simulink library "EOM_lib_incomplete"  (R2020a)
settings: Solver=VariableStepAuto  StartTime=0.0  StopTime=10.0  RelTol=1e-3
undefined symbols (not defined in the file or in its folder): g
libraries: $bdroot x1
settings Model: Creator=muril  LastModifiedBy=muril

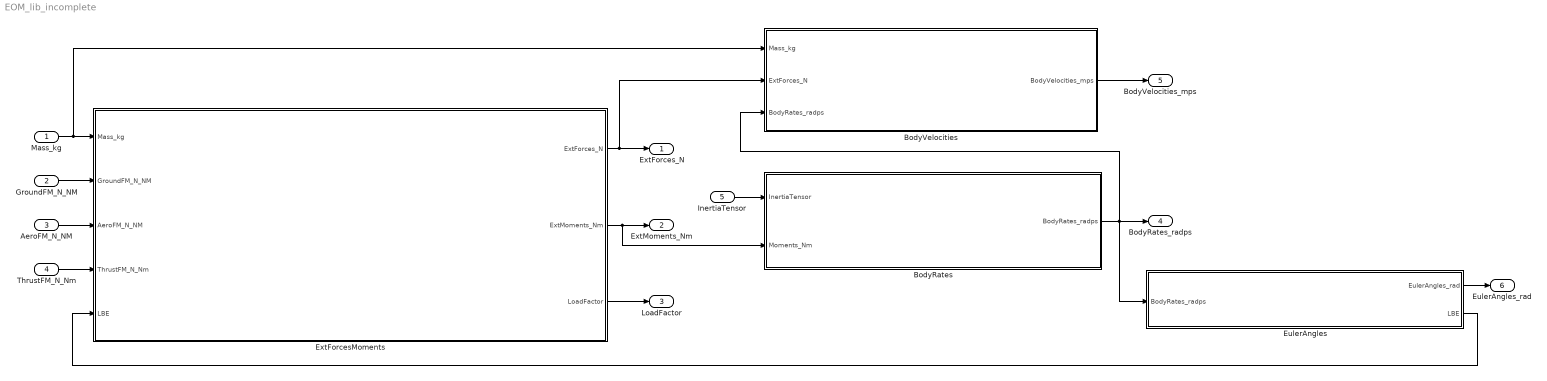
== system EOM_lib_incomplete ==
  Mass_kg : Inport
  GroundFM_N_NM : Inport  Port=2
  AeroFM_N_NM : Inport  Port=3
  ThrustFM_N_Nm : Inport  Port=4
  InertiaTensor : Inport  Port=5
  BodyRates : Subsystem
  BodyVelocities : Subsystem
  EulerAngles : Subsystem
  ExtForcesMoments : Subsystem
  ExtForces_N : Outport
  ExtMoments_Nm : Outport  Port=2
  LoadFactor : Outport  Port=3
  BodyRates_radps : Outport  Port=4
  BodyVelocities_mps : Outport  Port=5
  EulerAngles_rad : Outport  Port=6
  wires:
  EulerAngles/2(LBE) -> ExtForcesMoments/5(LBE)
  GroundFM_N_NM/1 -> ExtForcesMoments/2(GroundFM_N_NM)
  AeroFM_N_NM/1 -> ExtForcesMoments/3(AeroFM_N_NM)
  ThrustFM_N_Nm/1 -> ExtForcesMoments/4(ThrustFM_N_Nm)
  ExtForcesMoments/3(LoadFactor) -> LoadFactor/1
  InertiaTensor/1 -> BodyRates/1(InertiaTensor)
  ExtForcesMoments/2(ExtMoments_Nm) -> ExtMoments_Nm/1, BodyRates/2(Moments_Nm)
  BodyRates/1(BodyRates_radps) -> EulerAngles/1(BodyRates_radps), BodyRates_radps/1, BodyVelocities/3(BodyRates_radps)
  BodyVelocities/1(BodyVelocities_mps) -> BodyVelocities_mps/1
  ExtForcesMoments/1(ExtForces_N) -> BodyVelocities/2(ExtForces_N), ExtForces_N/1
  Mass_kg/1 -> BodyVelocities/1(Mass_kg), ExtForcesMoments/1(Mass_kg)
  EulerAngles/1(EulerAngles_rad) -> EulerAngles_rad/1

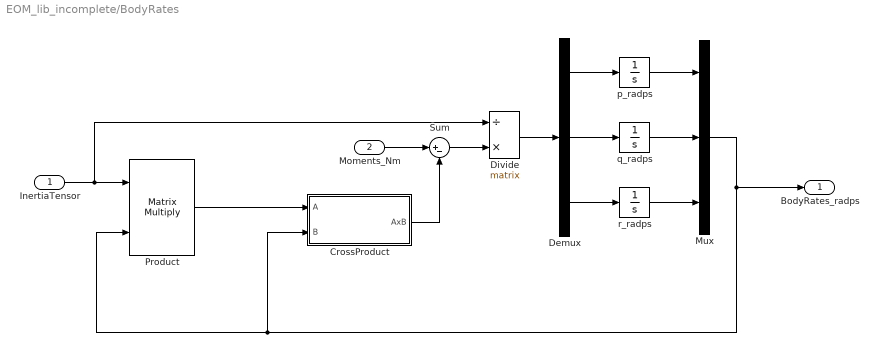
== system EOM_lib_incomplete/BodyRates ==
  InertiaTensor : Inport
  Moments_Nm : Inport  Port=2
  CrossProduct : Subsystem
  Demux : Demux  Outputs=3
  Divide : Product  Inputs=/*  Multiplication=Matrix(*)
  Mux : Mux  Inputs=3
  Product : Product  Multiplication=Matrix(*)
  Sum : Sum  Inputs=|+-
  p_radps : Integrator  ContinuousStateAttributes='p_radps'
  q_radps : Integrator  ContinuousStateAttributes='q_radps'
  r_radps : Integrator  ContinuousStateAttributes='r_radps'
  BodyRates_radps : Outport
  wires:
  Mux/1 -> BodyRates_radps/1, Product/2, CrossProduct/2(B)
  r_radps/1 -> Mux/3
  InertiaTensor/1 -> Product/1, Divide/1
  Product/1 -> CrossProduct/1(A)
  q_radps/1 -> Mux/2
  p_radps/1 -> Mux/1
  CrossProduct/1(AxB) -> Sum/2
  Demux/1 -> p_radps/1
  Sum/1 -> Divide/2
  Divide/1 -> Demux/1
  Moments_Nm/1 -> Sum/1
  Demux/2 -> q_radps/1
  Demux/3 -> r_radps/1

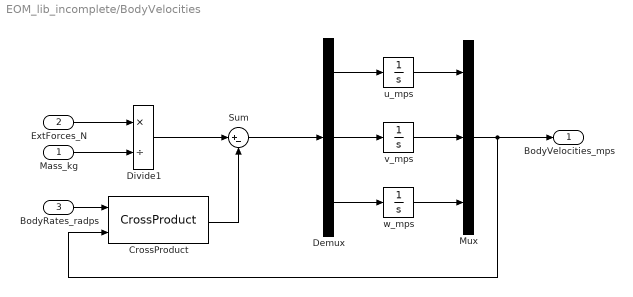
== system EOM_lib_incomplete/BodyVelocities ==
  Mass_kg : Inport
  ExtForces_N : Inport  Port=2
  BodyRates_radps : Inport  Port=3
  CrossProduct : $bdroot/BodyRates/CrossProduct  SystemSampleTime=-1  Latency=0  AutoFrameSizeCalculation=off
  Demux : Demux  Outputs=3
  Divide1 : Product  Inputs=*/
  Mux : Mux  Inputs=3
  Sum : Sum  Inputs=|+-
  u_mps : Integrator  ContinuousStateAttributes='u_mps'
  v_mps : Integrator  ContinuousStateAttributes='v_mps'
  w_mps : Integrator  ContinuousStateAttributes='w_mps'
  BodyVelocities_mps : Outport
  wires:
  BodyRates_radps/1 -> CrossProduct/1
  CrossProduct/1 -> Sum/2
  Demux/2 -> v_mps/1
  Demux/3 -> w_mps/1
  Divide1/1 -> Sum/1
  Demux/1 -> u_mps/1
  w_mps/1 -> Mux/3
  Mux/1 -> BodyVelocities_mps/1, CrossProduct/2
  u_mps/1 -> Mux/1
  Sum/1 -> Demux/1
  v_mps/1 -> Mux/2
  ExtForces_N/1 -> Divide1/1
  Mass_kg/1 -> Divide1/2

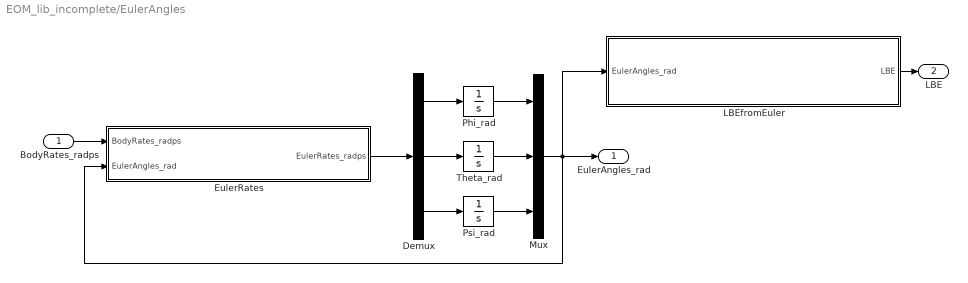
== system EOM_lib_incomplete/EulerAngles ==
  BodyRates_radps : Inport
  Demux : Demux  Outputs=3
  EulerRates : Subsystem
  LBEfromEuler : Subsystem
  Mux : Mux  Inputs=3
  Phi_rad : Integrator  ContinuousStateAttributes='Phi_rad'
  Psi_rad : Integrator  ContinuousStateAttributes='Psi_rad'
  Theta_rad : Integrator  ContinuousStateAttributes='Theta_rad'
  EulerAngles_rad : Outport
  LBE : Outport  Port=2
  wires:
  BodyRates_radps/1 -> EulerRates/1(BodyRates_radps)
  Demux/3 -> Psi_rad/1
  Theta_rad/1 -> Mux/2
  Psi_rad/1 -> Mux/3
  Mux/1 -> EulerRates/2(EulerAngles_rad), EulerAngles_rad/1, LBEfromEuler/1(EulerAngles_rad)
  Demux/1 -> Phi_rad/1
  Demux/2 -> Theta_rad/1
  Phi_rad/1 -> Mux/1
  EulerRates/1(EulerRates_radps) -> Demux/1
  LBEfromEuler/1(LBE) -> LBE/1

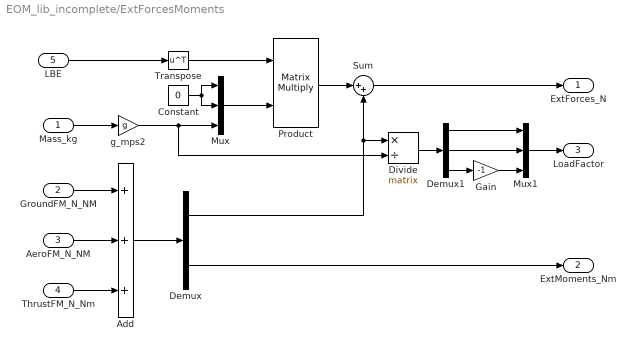
== system EOM_lib_incomplete/ExtForcesMoments ==
  Mass_kg : Inport
  GroundFM_N_NM : Inport  Port=2
  AeroFM_N_NM : Inport  Port=3
  ThrustFM_N_Nm : Inport  Port=4
  LBE : Inport  Port=5
  Add : Sum  Inputs=+++
  Constant : Constant  Value=0
  Demux : Demux  Outputs=2
  Demux1 : Demux  Outputs=3
  Divide : Product  Inputs=*/  Multiplication=Matrix(*)
  Gain : Gain  Gain=-1
  Mux : Mux  Inputs=3
  Mux1 : Mux  Inputs=3
  Product : Product  Multiplication=Matrix(*)
  Sum : Sum  Inputs=|++
  Transpose : Math  Operator=transpose  SaturateOnIntegerOverflow=on
  g_mps2 : Gain  Gain=g
  ExtForces_N : Outport
  ExtMoments_Nm : Outport  Port=2
  LoadFactor : Outport  Port=3
  wires:
  Demux/2 -> ExtMoments_Nm/1
  AeroFM_N_NM/1 -> Add/2
  Mux1/1 -> LoadFactor/1
  Constant/1 -> Mux/1, Mux/2
  Gain/1 -> Mux1/3
  Sum/1 -> ExtForces_N/1
  Demux/1 -> Divide/1, Sum/2
  ThrustFM_N_Nm/1 -> Add/3
  g_mps2/1 -> Divide/2, Mux/3
  GroundFM_N_NM/1 -> Add/1
  Add/1 -> Demux/1
  LBE/1 -> Transpose/1
  Demux1/3 -> Gain/1
  Mux/1 -> Product/2
  Mass_kg/1 -> g_mps2/1
  Transpose/1 -> Product/1
  Demux1/1 -> Mux1/1
  Product/1 -> Sum/1
  Demux1/2 -> Mux1/2
  Divide/1 -> Demux1/1

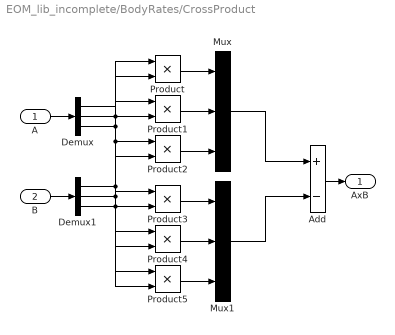
== system EOM_lib_incomplete/BodyRates/CrossProduct ==
  A : Inport
  B : Inport  Port=2
  Add : Sum  Inputs=+-
  Demux : Demux  Outputs=3
  Demux1 : Demux  Outputs=3
  Mux : Mux  Inputs=3
  Mux1 : Mux  Inputs=3
  Product{,1..5} (6 alike) : Product
  AxB : Outport
  wires:
  Demux1/1 -> Product5/2, Product1/2
  Mux1/1 -> Add/2
  Product1/1 -> Mux/2
  Product5/1 -> Mux1/3
  Demux/1 -> Product2/1, Product4/1
  Demux/3 -> Product3/1, Product1/1
  Demux/2 -> Product5/1, Product/1
  Demux1/2 -> Product3/2, Product2/2
  Product2/1 -> Mux/3
  A/1 -> Demux/1
  Product3/1 -> Mux1/1
  Add/1 -> AxB/1
  Demux1/3 -> Product4/2, Product/2
  Product/1 -> Mux/1
  Product4/1 -> Mux1/2
  Mux/1 -> Add/1
  B/1 -> Demux1/1

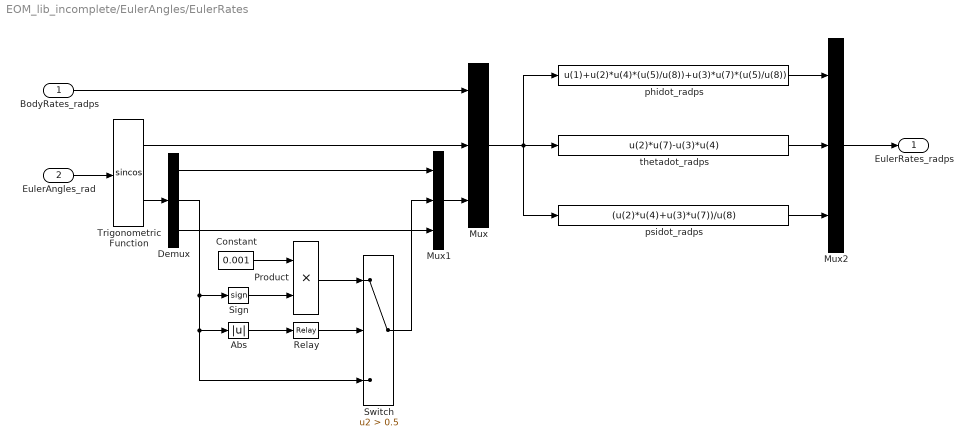
== system EOM_lib_incomplete/EulerAngles/EulerRates ==
  BodyRates_radps : Inport
  EulerAngles_rad : Inport  Port=2
  Abs : Abs
  Constant : Constant  Value=0.001
  Demux : Demux  Outputs=3
  Mux : Mux  Inputs=3
  Mux1 : Mux  Inputs=3
  Mux2 : Mux  Inputs=3
  Product : Product
  Relay : Relay  OnSwitchValue=0.001  OffSwitchValue=0  OnOutputValue=0  OffOutputValue=1
  Sign : Signum
  Switch : Switch  Criteria=u2 > Threshold  Threshold=0.5
  Trigonometric Function : Trigonometry  Operator=sincos
  phidot_radps : Fcn  Expr=u(1)+u(2)*u(4)*(u(5)/u(8))+u(3)*u(7)*(u(5)/u(8))
  psidot_radps : Fcn  Expr=(u(2)*u(4)+u(3)*u(7))/u(8)
  thetadot_radps : Fcn  Expr=u(2)*u(7)-u(3)*u(4)
  EulerRates_radps : Outport
  wires:
  Demux/3 -> Mux1/3
  Mux/1 -> psidot_radps/1, thetadot_radps/1, phidot_radps/1
  Trigonometric Function/1 -> Mux/2
  Mux2/1 -> EulerRates_radps/1
  BodyRates_radps/1 -> Mux/1
  Constant/1 -> Product/1
  Trigonometric Function/2 -> Demux/1
  Product/1 -> Switch/1
  EulerAngles_rad/1 -> Trigonometric Function/1
  psidot_radps/1 -> Mux2/3
  Demux/2 -> Abs/1, Switch/3, Sign/1
  Abs/1 -> Relay/1
  Demux/1 -> Mux1/1
  phidot_radps/1 -> Mux2/1
  Sign/1 -> Product/2
  Mux1/1 -> Mux/3
  Switch/1 -> Mux1/2
  Relay/1 -> Switch/2
  thetadot_radps/1 -> Mux2/2

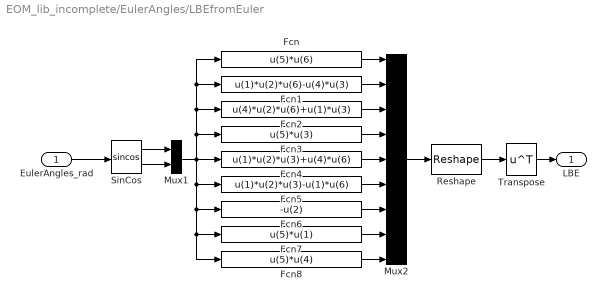
== system EOM_lib_incomplete/EulerAngles/LBEfromEuler ==
  EulerAngles_rad : Inport
  Fcn : Fcn  Expr=u(5)*u(6)
  Fcn1 : Fcn  Expr=u(1)*u(2)*u(6)-u(4)*u(3)
  Fcn2 : Fcn  Expr=u(4)*u(2)*u(6)+u(1)*u(3)
  Fcn3 : Fcn  Expr=u(5)*u(3)
  Fcn4 : Fcn  Expr=u(1)*u(2)*u(3)+u(4)*u(6)
  Fcn5 : Fcn  Expr=u(1)*u(2)*u(3)-u(1)*u(6)
  Fcn6 : Fcn  Expr=-u(2)
  Fcn7 : Fcn  Expr=u(5)*u(1)
  Fcn8 : Fcn  Expr=u(5)*u(4)
  Mux1 : Mux  Inputs=2
  Mux2 : Mux  Inputs=9
  Reshape : Reshape  OutputDimensionality=Customize  OutputDimensions=[3,3]
  SinCos : Trigonometry  Operator=sincos
  Transpose : Math  Operator=transpose  SaturateOnIntegerOverflow=on
  LBE : Outport
  wires:
  Fcn6/1 -> Mux2/7
  Reshape/1 -> Transpose/1
  SinCos/2 -> Mux1/2
  Fcn/1 -> Mux2/1
  Fcn2/1 -> Mux2/3
  Mux2/1 -> Reshape/1
  Fcn7/1 -> Mux2/8
  Fcn1/1 -> Mux2/2
  Mux1/1 -> Fcn8/1, Fcn7/1, Fcn6/1, Fcn5/1, Fcn/1, Fcn1/1, Fcn2/1, Fcn3/1, Fcn4/1
  Fcn3/1 -> Mux2/4
  Fcn5/1 -> Mux2/6
  Fcn8/1 -> Mux2/9
  Fcn4/1 -> Mux2/5
  SinCos/1 -> Mux1/1
  Transpose/1 -> LBE/1
  EulerAngles_rad/1 -> SinCos/1
